simulink model "step_Bridg"  (Simulink 8.8)
settings: Solver=ode45  StartTime=0.0  StopTime=30  MaxStep=0.1  RelTol=1e-3  EnableMultiTasking=on
values from neighbouring files (symbols this model uses):
  Dm = str2double(get(handles.Dm,'string'))    [tgb.m]
  g = 9.8    [tgb.m]
  K = str2double(get(handles.K,'string'))    [tgb.m]
  KK = lqr(A,B,Q,R)    [tgb.m]
  l = 20    [drow_wt.m]    (also in tgb.m = str2double(get(handles.l,'string')))
  Td = str2double(get(handles.Td,'string'))    [tgb.m]
  Wm = str2double(get(handles.Wm,'string'))    [tgb.m]
  X_0 = 100/3*X_0    (= 3333.33333333)    [tgb.m]
settings Model: Creator=Administrator  LastModifiedBy=WIN10
settings DataIOCC: SignalLoggingSaveFormat=Dataset  OutputSaveName=y1,y2,y3,y4,y5
settings OptimizationCC: ExpressionDepthLimit=2147483647
settings DebuggingCC: FcnCallInpInsideContextMsg=error
settings GRTTargetCC: CombineOutputUpdateFcns=on  GRTInterface=off
settings ConfigComp: CovSFcnEnable=off

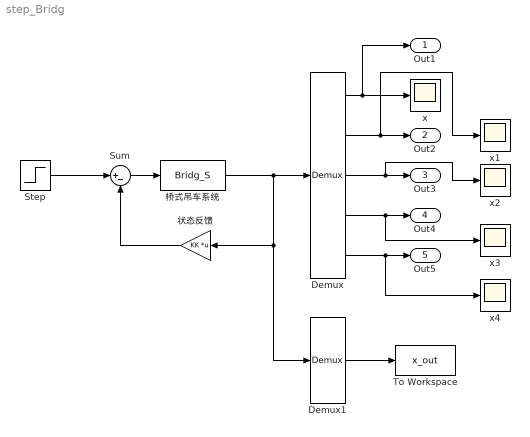
== system step_Bridg ==
  Demux : Demux  Outputs=5
  Demux1 : Demux  Outputs=1
  Step : Step  Time=0  After=10  SampleTime=0
  Sum : Sum  Inputs=|+-
  To Workspace : ToWorkspace  VariableName=x_out  SaveFormat=Structure With Time  SampleTime=-1
  x{,1..4} (5 alike) : Scope
  桥式吊车系统 : S-Function  FunctionName=Bridg_S  Parameters=Dm,Wm,l,K,Td,g,X_0  SFunctionDeploymentMode=off  EnableBusSupport=off  mask(***桥式吊车系统参数设置***){Dm=Dm, wm=Wm, l=l, K=K, Td=Td, g=g, X_0=X_0}
      mask prompts: Dm "吊车质量"; wm "物体质量"; l "绳子的长度"; K "电压驱动放大"; Td "电机时间常数"; g "重力加速度"; X_0 "预定到达的水平位置"
      mask help: This is a bridge crane system. You can set the following parameters:
      mask Display: disp('桥式吊车系统')
  状态反馈 : Gain  Gain=KK  Multiplication=Matrix(K*u)
  Out1 : Outport
  Out2 : Outport  Port=2
  Out3 : Outport  Port=3
  Out4 : Outport  Port=4
  Out5 : Outport  Port=5
  wires:
  桥式吊车系统/1 -> 状态反馈/1, Demux1/1, Demux/1
  Demux/1 -> Out1/1, x/1
  Demux/2 -> x1/1, Out2/1
  Demux/3 -> x2/1, Out3/1
  Demux1/1 -> To Workspace/1
  Sum/1 -> 桥式吊车系统/1
  Demux/4 -> x3/1, Out4/1
  Demux/5 -> x4/1, Out5/1
  Step/1 -> Sum/1
  状态反馈/1 -> Sum/2
